simulink model "discrete_LQR_control"  (R2023b)
settings: Solver=FixedStepAuto  StartTime=0.0  StopTime=40  FixedStep=0.002  RelTol=1e-3  EnableMultiTasking=on
InitFcn:
  | %run('C:\Users\Jonathan de Brusse\Desktop\QuanserQube2 - research\Control of the pendulum\Discounted_LQR_analysis.m')
  | run('C:\Users\Jonathan de Brusse\Desktop\QuanserQube2 - research\Control of the pendulum\control_balance_reduced_order.m')
  | %run('C:\Users\Jonathan de Brusse\Desktop\QuanserQube2 - research\Control of the pendulum\Data_driven.m')
values from neighbouring files (symbols this model uses):
  calib_time = 5    [control_balance_reduced_order.m]    (also in qube_system_params.m)
  Kv = Yv*inv(Gv)    [control_balance_reduced_order.m]
undefined symbols (not defined in the file or in its folder): HIL, qc_get_step_size
libraries: quarc_library x9
settings Model: ExtModeTrigDuration=10000  Creator=Jonathan de Brusse  LastModifiedBy=Jonathan de Brusse
settings SolverCC: AlgebraicLoopSolver=TrustRegion  PositivePriorityOrder=on
settings DataIOCC: ReturnWorkspaceOutputs=off
settings DebuggingCC: UnconnectedInputMsg=warning  UnconnectedOutputMsg=warning  UnconnectedLineMsg=warning  ArithmeticOperatorsInVariantConditions=warning
settings ModelReferenceCC: EnableRefExpFcnMdlSchedulingChecks=on
settings SFSimCC: SimUseLocalCustomCode=off  CustomCodeUndefinedFunction=UseInterfaceOnly
settings RTWCC: Description=QUARC Win64 Target Using Toolchain  SystemTargetFile=quarc_win64.tlc  TemplateMakefile=quarc_default_tmf  RTWUseLocalCustomCode=off  Toolchain=QUARC win64 | nmake (64-bit Windows)  BuildConfiguration=Faster Runs
settings CodeAppCC: StateflowObjectComments=on
settings STFCustomTargetCC: ConcurrentExecutionCompliant=on  GRTInterface=on  UseToolchainInfoCompliant=on  SystemTargetFile=quarc_win64.tlc
settings GRTTargetCC: ParMdlRefBuildCompliant=off  CompOptLevelCompliant=off  CombineOutputUpdateFcns=off  MatFileLogging=off  CPPClassGenCompliant=off  GRTInterface=on  ExtMode=on  ExtModeMexFile=quarc_comm
settings ConfigComp: CovMetricSettings=dswe

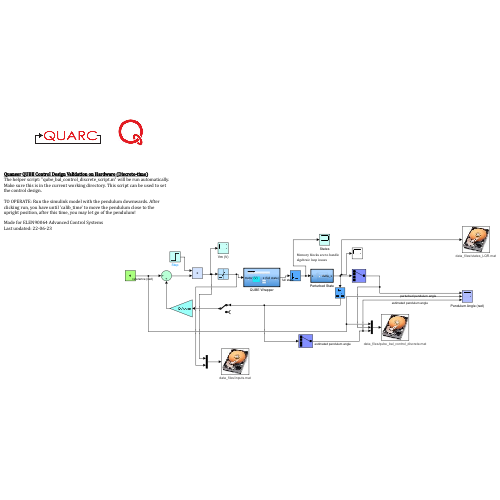
[thumbnail: Simulink's stored preview of the top-level diagram]
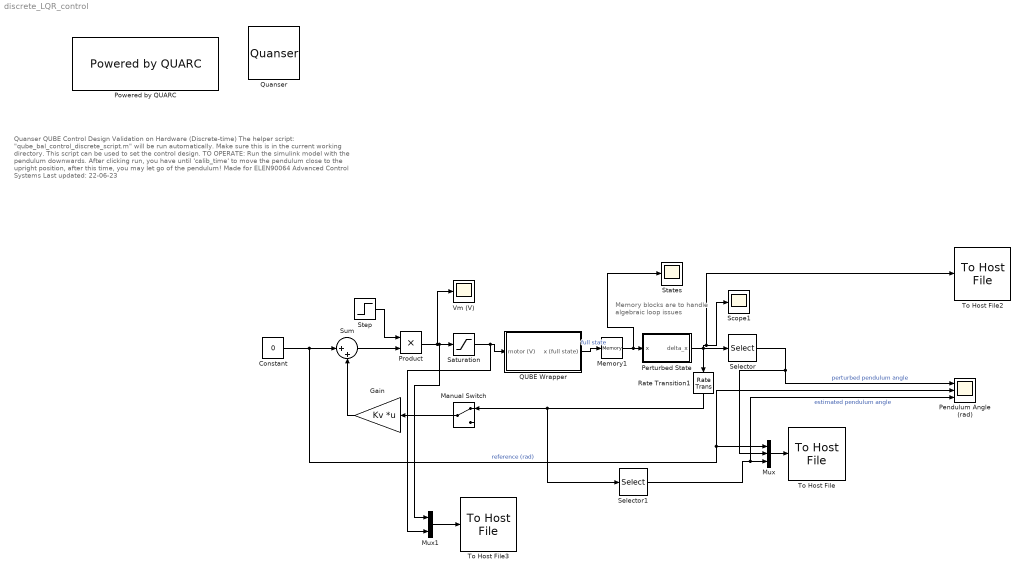
== system discrete_LQR_control ==
  note: Quanser QUBE Control Design Validation on Hardware (Discrete-time)
      | The helper script: "qube_bal_control_discrete_script.m" will be run automatically. Make sure this is in the current working directory. This script can be used to set the control design.
      |
      | TO OPERATE: Run the simulink model with the pendulum downwards. After clicking run, you have until 'calib_time' to move the pendulum close to the upright position, after this time, you may let go of the pendulum!
      |
      | Made for ELEN90064 Advanced Control Systems
      | Last updated: 22-06-23
  note: Memory blocks are to handle
      | algebraic loop issues
  Constant : Constant  Value=0  SampleTime=-1
  Gain : Gain  Gain=Kv  Multiplication=Matrix(K*u) (u vector)
  Manual Switch : ManualSwitch
  Memory1 : Memory
  Mux : Mux  Inputs=3
  Mux1 : Mux  Inputs=2
  Pendulum Angle (rad) : Scope  NumInputPorts=3
  Perturbed State : Subsystem  TreatAsAtomicUnit=on
  Powered by QUARC : quarc_library/Logos/Powered by QUARC
  Product : Product
  QUBE Wrapper : Subsystem  TreatAsAtomicUnit=on
  Quanser : quarc_library/Logos/Quanser
  Rate Transition1 : RateTransition  OutPortSampleTime=delta
  Saturation : Saturate  UpperLimit=10  LowerLimit=-10
  Scope1 : Scope
  Selector : Selector  InputPortWidth=4  IndexOptions=Index vector (dialog)  Indices=[1]  OutputSizes=1
  Selector1 : Selector  InputPortWidth=4  IndexOptions=Index vector (dialog)  Indices=[1]  OutputSizes=1
  States : Scope
  Step : Step  Time=calib_time  SampleTime=0
  Sum : Sum  Inputs=|++
  To Host File : quarc_library/Sinks/To Host/To Host File  file_name=data_files/qube_bal_control_discrete.mat  variable_name=outputs  decimation=1  sample_time=-1  file_format=MAT-file v.4  options=No header or footer  append=off  final_file_name=data_files/qube_bal_control_discrete.mat  bitrate=2000000
  To Host File2 : quarc_library/Sinks/To Host/To Host File  file_name=data_files/states_LQR.mat  variable_name=data  decimation=1  sample_time=-1  file_format=MAT-file v.4  options=No header or footer  append=off  final_file_name=data_files/states_LQR.mat  bitrate=2000000
  To Host File3 : quarc_library/Sinks/To Host/To Host File  file_name=data_files/inputs.mat  variable_name=data  decimation=1  sample_time=-1  file_format=MAT-file v.4  options=No header or footer  append=off  final_file_name=data_files/inputs.mat  bitrate=2000000
  Vm (V) : Scope
  wires:
  Perturbed State/1(delta_x) -> To Host File2/1, Scope1/1, Selector/1, Rate Transition1/1
  Product/1 -> Mux1/1, Saturation/1, Vm (V)/1
  Memory1/1 -> States/1, Perturbed State/1(x)
  Step/1 -> Product/1
  Rate Transition1/1 -> Selector1/1, Manual Switch/1
  Sum/1 -> Product/2
  Mux/1 -> To Host File/1
  Constant/1 -> Sum/1, Pendulum Angle (rad)/2, Mux/1  "reference (rad)"
  Saturation/1 -> Mux1/2, QUBE Wrapper/1(motor (V))
  QUBE Wrapper/1(x (full state)) -> Memory1/1  "full state"
  Gain/1 -> Sum/2
  Selector/1 -> Mux/2, Pendulum Angle (rad)/1  "perturbed pendulum angle"
  Selector1/1 -> Pendulum Angle (rad)/3, Mux/3  "estimated pendulum angle"
  Manual Switch/1 -> Gain/1
  Mux1/1 -> To Host File3/1

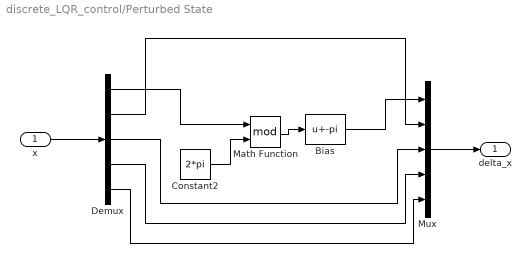
== system discrete_LQR_control/Perturbed State ==
  x : Inport
  Bias : Bias  Bias=-pi  SaturateOnIntegerOverflow=off
  Constant2 : Constant  Value=2*pi
  Demux : Demux  Outputs=5
  Math Function : Math  Operator=mod  SignedPower=on
  Mux : Mux  Inputs=5
  delta_x : Outport  VectorParamsAs1DForOutWhenUnconnected=off
  wires:
  Math Function/1 -> Bias/1
  Constant2/1 -> Math Function/2
  x/1 -> Demux/1
  Demux/3 -> Mux/3
  Demux/4 -> Mux/4
  Mux/1 -> delta_x/1
  Demux/5 -> Mux/5
  Demux/1 -> Math Function/1
  Bias/1 -> Mux/1
  Demux/2 -> Mux/2

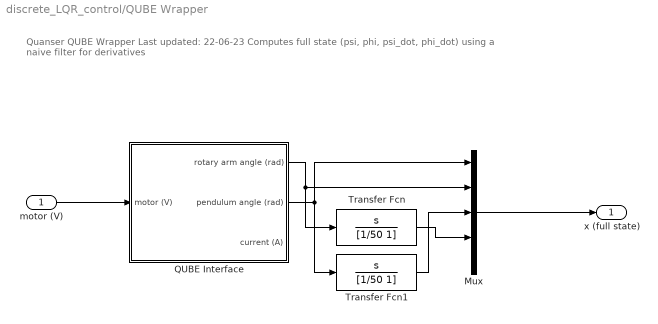
== system discrete_LQR_control/QUBE Wrapper ==
  note: Quanser QUBE Wrapper
      | Last updated: 22-06-23
      | Computes full state (psi, phi, psi_dot, phi_dot) using a naive filter for derivatives
  motor (V) : Inport
  Mux : Mux  Inputs=5
  QUBE Interface : Subsystem
  Transfer Fcn : TransferFcn  Numerator=[1 0]  Denominator=[1/50 1]
  Transfer Fcn1 : TransferFcn  Numerator=[1 0]  Denominator=[1/50 1]
  x (full state) : Outport  VectorParamsAs1DForOutWhenUnconnected=off
  wires:
  motor (V)/1 -> QUBE Interface/1(motor (V))
  QUBE Interface/1(rotary arm angle (rad)) -> Mux/2, Transfer Fcn/1
  QUBE Interface/2(pendulum angle (rad)) -> Transfer Fcn1/1, Mux/1
  Mux/1 -> x (full state)/1
  Transfer Fcn/1 -> Mux/4
  Transfer Fcn1/1 -> Mux/3

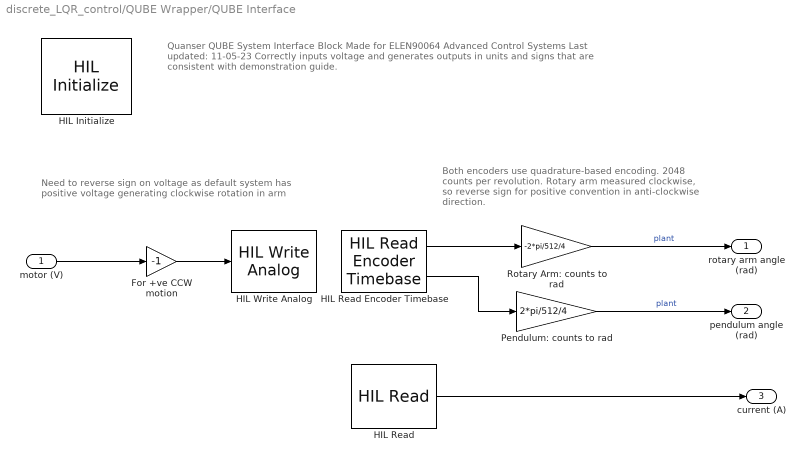
== system discrete_LQR_control/QUBE Wrapper/QUBE Interface ==
  note: Need to reverse sign on voltage as default system has
      | positive voltage generating clockwise rotation in arm
  note: Quanser QUBE System Interface Block
      | Made for ELEN90064 Advanced Control Systems
      | Last updated: 11-05-23
      |
      | Correctly inputs voltage and generates outputs in units and signs that
      | are consistent with demonstration guide.
  note: Both encoders use quadrature-based encoding.
      | 2048 counts per revolution.
      | Rotary arm measured clockwise, so reverse sign for
      | positive convention in anti-clockwise direction.
  motor (V) : Inport  OutDataTypeStr=double  PortDimensions=1
  For +ve CCW motion : Gain  Gain=-1
  HIL Initialize : quarc_library/Data Acquisition/Generic/Configuration/HIL Initialize  object_name=HIL-1  board_type=qube_servo2_usb  board_number=0  board_options=""  exclusive=off  active=on  hardware_clocks=[0]  clock_modes=[]  initial_clock_frequencies=[]  set_clock_params_at_start=off  set_clock_params_at_switch_in=off  set_clock_frequencies_at_start=off  set_clock_frequencies_at_switch_in=off  analog_input_channels=[0]  analog_input_configurations=[]  analog_input_maximums=3  analog_input_minimums=-3  set_analog_input_params_at_start=off  set_analog_input_params_at_switch_in=off  analog_output_channels=[0]  analog_output_maximums=15  analog_output_minimums=-15  initial_analog_outputs=[0]  final_analog_outputs=[0]  watchdog_analog_outputs=0  set_analog_output_params_at_start=off  set_analog_output_params_at_switch_in=off  set_analog_outputs_at_start=on  set_analog_outputs_at_switch_in=off  set_analog_outputs_at_terminate=on  set_analog_outputs_at_switch_out=off  set_analog_outputs_on_watchdog=on  digital_input_channels=[]  digital_output_channels=[0]  digital_output_configuration=[]  initial_digital_outputs=[1]  final_digital_outputs=[0]  watchdog_digital_outputs=[0]  set_digital_output_params_at_start=off  set_digital_output_params_at_switch_in=off  set_digital_outputs_at_start=on  set_digital_outputs_at_switch_in=off  set_digital_outputs_at_terminate=on  set_digital_outputs_at_switch_out=off  set_digital_outputs_on_watchdog=on  encoder_channels=[0:1]  quadrature=[4]  encoder_filter_frequency=[]  initial_encoder_counts=[0]  set_encoder_params_at_start=off  set_encoder_params_at_switch_in=off  set_encoder_counts_at_start=on  set_encoder_counts_at_switch_in=off  pwm_channels=[]  pwm_modes=[]  pwm_frequency=[]  pwm_configuration=[]  pwm_alignment=[]  pwm_polarity=[]  pwm_leading_deadband=[]  pwm_trailing_deadband=[]  initial_pwm_outputs=[]  final_pwm_outputs=[]  watchdog_pwm_outputs=[]  set_pwm_params_at_start=off  set_pwm_params_at_switch_in=off  set_pwm_outputs_at_start=off  set_pwm_outputs_at_switch_in=off  set_pwm_outputs_at_terminate=off  set_pwm_outputs_at_switch_out=off  set_pwm_outputs_on_watchdog=off  other_output_channels=[11000:11002]  initial_other_outputs=[0 1 0]  final_other_outputs=[1 0 0]  watchdog_other_outputs=[0 0 1]  set_other_outputs_at_start=on  set_other_outputs_at_switch_in=off  set_other_outputs_at_terminate=on  set_other_outputs_at_switch_out=off  set_other_outputs_on_watchdog=on
  HIL Read : quarc_library/Data Acquisition/Generic/Immediate I//O/HIL Read  object_name=HIL-1  analog_channels=0  encoder_channels=[]  digital_channels=[]  other_channels=[]  sample_time=qc_get_step_size  active=on  vector_output=off  data_type_mode=Inherit via back propagation  encoder_data_type=double  digital_data_type=boolean
  HIL Read Encoder Timebase : quarc_library/Data Acquisition/Generic/Timebases/HIL Read Encoder Timebase  object_name=HIL-1  clock=0  channels=[0,1]  active=on  vector_output=off  data_type_mode=Inherit via back propagation  data_type=double  overflow_mode=Error on overflow  samples_in_buffer=max(ceil(1/qc_get_step_size), 1)
  HIL Write Analog : quarc_library/Data Acquisition/Generic/Immediate I//O/HIL Write Analog  object_name=HIL-1  channels=0  sample_time=-1  active=off  vector_input=off
  Pendulum: counts to rad : Gain  Gain=2*pi/512/4
  Rotary Arm: counts to rad : Gain  Gain=-2*pi/512/4
  rotary arm angle (rad) : Outport  OutDataTypeStr=double  PortDimensions=1  SampleTime=[0.002,0]  VectorParamsAs1DForOutWhenUnconnected=off
  pendulum angle (rad) : Outport  Port=2  OutDataTypeStr=double  PortDimensions=1  SampleTime=[0.002,0]  VectorParamsAs1DForOutWhenUnconnected=off
  current (A) : Outport  Port=3
  wires:
  For +ve CCW motion/1 -> HIL Write Analog/1
  motor (V)/1 -> For +ve CCW motion/1
  Pendulum: counts to rad/1 -> pendulum angle (rad)/1  "plant"
  HIL Read Encoder Timebase/1 -> Rotary Arm: counts to rad/1
  Rotary Arm: counts to rad/1 -> rotary arm angle (rad)/1  "plant"
  HIL Read Encoder Timebase/2 -> Pendulum: counts to rad/1
  HIL Read/1 -> current (A)/1
